simulink model "liveness"  (R2021b)
settings: Solver=FixedStepAuto  StartTime=0.0  StopTime=10.0  RelTol=1e-3
undefined symbols (not defined in the file): sldvsubsys
libraries: sldvlib x9, simulink x2
settings Model: Creator=marco  LastModifiedBy=angelo
settings ConfigComp: DVMode=PropertyProving  DVTestSuiteOptimization=Auto  DVDetectOutOfBounds=on  DVProvingStrategy=FindViolation  DVModelReferenceHarness=on

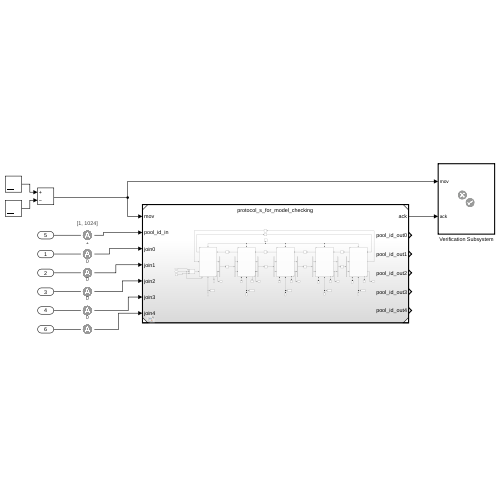
[thumbnail: Simulink's stored preview of the top-level diagram]
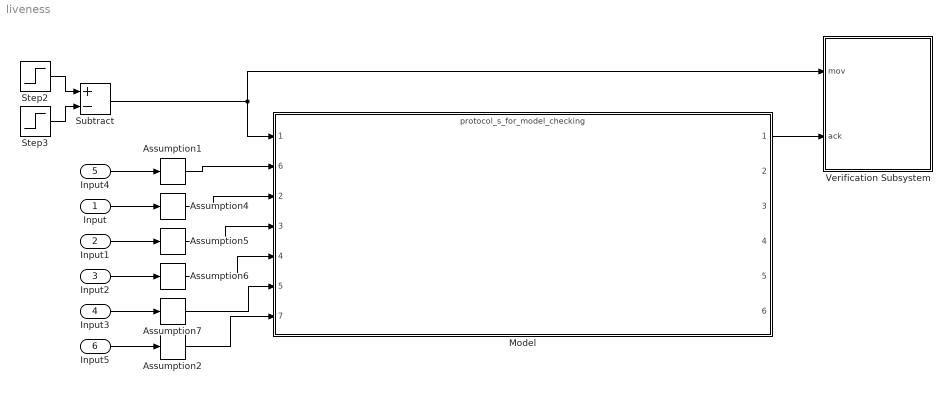
== system liveness ==
  Input : Inport
  Input1 : Inport  Port=2
  Input2 : Inport  Port=3
  Input3 : Inport  Port=4
  Input4 : Inport  Port=5
  Input5 : Inport  Port=6
  Assumption1 : sldvlib/Objectives and Constraints/Assumption  enabled=on  customAVTBlockType=Assumption  intervals=[1, 1024]  initial=off  dispValues=on  outEnabled=on
      settings: AttributesFormatString=%<intervals>  SourceProductBaseCode=SL
  Assumption{2,5..7} (4 alike) : sldvlib/Objectives and Constraints/Assumption  enabled=on  customAVTBlockType=Assumption  intervals=0  initial=off  dispValues=on  outEnabled=on
      settings: AttributesFormatString=%<intervals>  SourceProductBaseCode=SL
  Assumption4 : sldvlib/Objectives and Constraints/Assumption  enabled=on  customAVTBlockType=Assumption  intervals=1  initial=off  dispValues=on  outEnabled=on
      settings: AttributesFormatString=%<intervals>  SourceProductBaseCode=SL
  Model : ModelReference  ModelNameDialog=protocol_s_for_model_checking.slx  SimulationMode=Normal  ModelReferenceVersion=1.126
      settings: PortSchema="{\"entries\":[{\"content\":{\"sides\":[{\"content\":{\"connectorIds\":[\"In1\",\"In6\",\"In2\",\"In3\",\"In4\",\"In5\",\"In7\"]},\"type\":\"ConnectorPlacement.EquallySpacedRectSide\",\"uuid\":\"2cc34edd-a176-40cb-b6fa-8cbf6e460119\"},{\"content\":{\"connectorIds\":[\"Out1\",\"Out2\",\"Out3\",\"Out4\",\"Out5\",\"Out6\"],\"side\":\"RIGHT\"},\"type\":\"ConnectorPlacement.EquallySpacedRectSide\",\"uuid\":\"b9fb4b35-80b7-4954-be48-a4c9e0c81b3a\"},{\"content\":{\"connectorIds\":[],\"side\":\"TOP\"},\"type\":\"ConnectorPlacement.EquallySpacedRectSide\",\"uuid\":\"9d4ba344-f407-4b95-9191-bce6cbc03920\"}]},\"type\":\"ConnectorPlacement.EquallySpacedConnector\",\"uuid\":\"c770100c-051e-4872-aa3a-ba047be3662c\"}],\"packageUris\":[\"http://schema.mathworks.com/mf0/Connector/R2020b\"],\"version\":\"1.0\"}"
  Step2 : Step  SampleTime=.2
  Step3 : Step  Time=1.2  SampleTime=.2
  Subtract : Sum  Inputs=+-
  Verification Subsystem : Subsystem  Tag=VerificationSubsystem  DisableCoverage=on  LoadFcn=sldvsubsys('check')  TreatAsAtomicUnit=on  SimViewingDevice=on  mask(VerificationSubsystem){}
      mask init:
      | sldvsubsys('maskInit');
      settings: CopyFcn=sldvsubsys('copy');  OpenFcn=open_system(gcb,'force');
      settings: PreSaveFcn=|
      | set_param(gcb,'SimViewingDevice','on');
      | sldvsubsys('check');
      mask Help: helpview(fullfile(docroot,'toolbox','sldv','sldv.map'),'verificationsubsystem')
      mask Display: image(imread('sldvicon_versubsys.png','BackGroundColor',[1 1 1]),'center');
  wires:
  Step2/1 -> Subtract/1
  Step3/1 -> Subtract/2
  Subtract/1 -> Model/1, Verification Subsystem/1(mov)
  Assumption4/1 -> Model/2
  Assumption5/1 -> Model/3
  Assumption6/1 -> Model/4
  Assumption7/1 -> Model/5
  Model/1 -> Verification Subsystem/2(ack)
  Assumption1/1 -> Model/6
  Input/1 -> Assumption4/1
  Input3/1 -> Assumption7/1
  Input2/1 -> Assumption6/1
  Input1/1 -> Assumption5/1
  Input4/1 -> Assumption1/1
  Input5/1 -> Assumption2/1
  Assumption2/1 -> Model/7

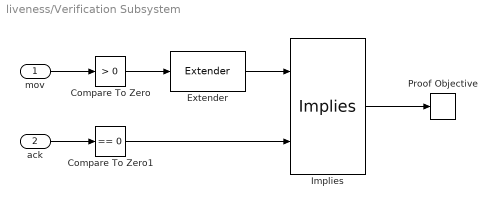
== system liveness/Verification Subsystem ==
  mov : Inport
  ack : Inport  Port=2
  Compare To Zero : simulink/Logic and Bit Operations/Compare To Zero  relop=>  OutDataTypeStr=boolean
  Compare To Zero1 : simulink/Logic and Bit Operations/Compare To Zero  relop===  OutDataTypeStr=boolean
  Extender : sldvlib/Temporal Operators/Extender  reset=off  ext_type=Infinite  out_hold=3
      settings: SourceProductBaseCode=SL
  Implies : sldvlib/Verification Utilities/Implies
      settings: SourceProductBaseCode=SL
  Proof Objective : sldvlib/Objectives and Constraints/Proof Objective  enabled=on  customAVTBlockType=Proof Objective  intervals=true  dispValues=on  outEnabled=off  enableStopSim=off
      settings: AttributesFormatString=%<intervals>  SourceProductBaseCode=SL
  wires:
  ack/1 -> Compare To Zero1/1
  Compare To Zero1/1 -> Implies/2
  Implies/1 -> Proof Objective/1
  mov/1 -> Compare To Zero/1
  Compare To Zero/1 -> Extender/1
  Extender/1 -> Implies/1
